simulink model "Controlled_FullWave_ConstantCurrent"  (R2021a)
settings: Solver=VariableStepAuto  StartTime=0.0  StopTime=0.8  MaxStep=1e-6  RelTol=1e-3
libraries: spsThyristorLib x4, spsACVoltageSourceLib x1, spsControlledCurrentSourceLib x1, spsMeanLib x1, spsVoltageMeasurementLib x1, spspowerguiLib x1
settings Model: Creator=Shashwat M.A  LastModifiedBy=Shashwat M.A

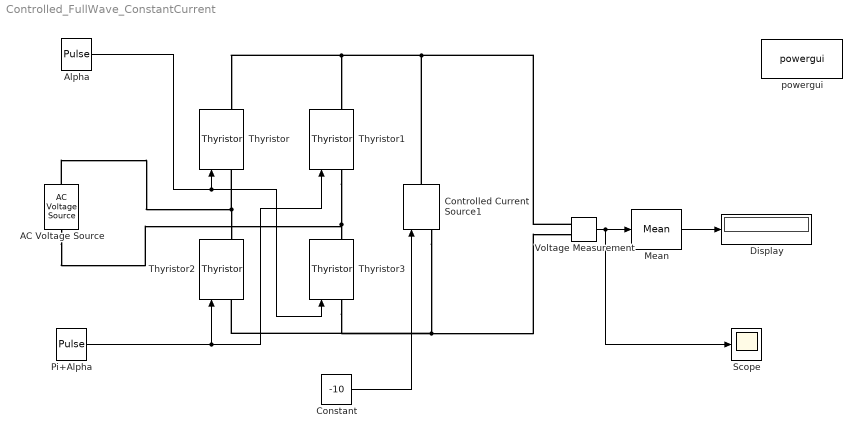
== system Controlled_FullWave_ConstantCurrent ==
  AC Voltage Source : spsACVoltageSourceLib/AC Voltage Source  Amplitude=325  Phase=0  Frequency=50  SampleTime=0  Measurements=None  BusType=swing  Pref=10e3  Qref=0  Qmin=-inf  Qmax=+inf
  Alpha : DiscretePulseGenerator  PulseType=Time based  Period=0.02  PulseWidth=5  PhaseDelay=120/360*0.02
  Constant : Constant  Value=-10
  Controlled Current Source1 : spsControlledCurrentSourceLib/Controlled Current Source  Initialize=on  Source_Type=AC  Amplitude=0  Phase=0  Frequency=0  Measurements=None
  Display : Display
  Mean : spsMeanLib/Mean  Freq=50  Vinit=0  Ts=0
  Pi+Alpha : DiscretePulseGenerator  PulseType=Time based  Period=0.02  PulseWidth=5  PhaseDelay=300/360*0.02
  Scope : Scope
  Thyristor{,1..3} (4 alike) : spsThyristorLib/Thyristor  Ron=0.001  Lon=0  Vf=0.8  IC=0  Rs=500  Cs=250e-9  Measurements=on
  Voltage Measurement : spsVoltageMeasurementLib/Voltage Measurement  PhasorSimulation=off  OutputType=Complex  PSBequivalent=0
  powergui : spspowerguiLib/powergui  Priority=1  SimulationMode=Continuous  SampleTime=50e-6  frequency=60  Iterations=50  frequencyindice=50  Pbase=100e6  ErrMax=1e-4  UnitsV=kV  UnitsW=MW  buscounter=0  FunctionMessages=off  echomessages=off  EnableUseOfTLC=off  CurrentSourceSwitches=off  DisableSnubberDevices=off  DisableRonSwitches=off  DisableVfSwitches=off  DisplayEquations=off  AutomaticDiscreteSolvers=off  SolverType=Tustin/Backward Euler (TBE)  Interpol=off  ExternalGateDelay=off  methode=off  Ts=100  x0status=blocks  SPID=on  SwTol=0  HookPort=off  NonlinearTolerance=1e-4  nMaxIteration=100  ContinueOnMaxIteration=off  RestoreLinks=warning  ResistiveCurrentMeasurement=off  Frange=[0:2:500]  Ylog=off  Xlog=on  ShowGrid=off  save=off  variable=ZData  structure=0  ZoomFFT=off  StartTime=0.0  cycles=1  DisplayStyle=1  fundamental=60  FreqAxis=off  MaxFrequency=1000  frequencyindicesteady=1  RmsSteady=1  display=off
  wires:
  Voltage Measurement/1 -> Scope/1, Mean/1
  Mean/1 -> Display/1
  Alpha/1 -> Thyristor3/1, Thyristor/1
  Pi+Alpha/1 -> Thyristor1/1, Thyristor2/1
  Constant/1 -> Controlled Current Source1/1
  connections:
  AC Voltage Source/RConn1 -- Thyristor2/RConn1 -- Thyristor/LConn1
  AC Voltage Source/LConn1 -- Thyristor1/LConn1 -- Thyristor3/RConn1
  Voltage Measurement/LConn1 -- Controlled Current Source1/RConn1 -- Thyristor1/RConn1 -- Thyristor/RConn1
  Thyristor3/LConn1 -- Thyristor2/LConn1 -- Controlled Current Source1/LConn1 -- Voltage Measurement/LConn2
